simulink model "steady_state"  (R2018b)
settings: Solver=FixedStepAuto  StartTime=0.0  StopTime=0.9  FixedStep=1e-6  RelTol=1e-3
values from neighbouring files (symbols this model uses):
  J = 0.09    [dq_3hp_induction.m]
  load_time = 0.5    [dq_3hp_induction.m]
  P = 4    [dq_3hp_induction.m]
  rrp = 0.8    [dq_3hp_induction.m]
  rs = 0.45    [dq_3hp_induction.m]
  v_ll = v_rms/sqrt(3)    [dq_3hp_induction.m]
  wb = 2*pi*f    (= 376.991118431)    [dq_3hp_induction.m]
  X_lr_p = 0.75    [dq_3hp_induction.m]
  X_ls = 0.75    [dq_3hp_induction.m]
  X_M = 27    [dq_3hp_induction.m]
libraries: simulink_extras x7
settings Model: Creator=carlo  LastModifiedBy=carlo

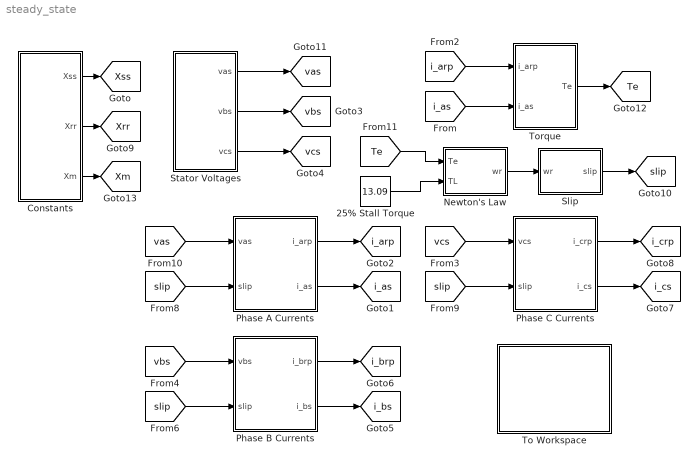
== system steady_state ==
  25% Stall Torque : Constant  Value=13.09
  Constants : Subsystem
  Newton's Law : Subsystem
  Phase A Currents : Subsystem
  Phase B Currents : Subsystem
  Phase C Currents : Subsystem
  Slip : Subsystem
  Stator Voltages : Subsystem
  To Workspace : Subsystem
  Torque : Subsystem
  tag scope: Te=global, Xm=global, Xrr=global, Xss=global, i_arp=global, i_as=global, i_brp=global, i_bs=global, i_crp=global, i_cs=global, slip=global, vas=global, vbs=global, vcs=global
  wires:
  Newton's Law/1(wr) -> Slip/1(wr)
  Slip/1(slip) -> [slip]
  [vas] -> Phase A Currents/1(vas)
  [slip] -> Phase A Currents/2(slip)
  Phase A Currents/1(i_arp) -> [i_arp]
  Phase A Currents/2(i_as) -> [i_as]
  [i_arp] -> Torque/1(i_arp)
  [i_as] -> Torque/2(i_as)
  Torque/1(Te) -> [Te]
  [Te] -> Newton's Law/1(Te)
  Stator Voltages/1(vas) -> [vas]
  Stator Voltages/2(vbs) -> [vbs]
  Stator Voltages/3(vcs) -> [vcs]
  Phase B Currents/1(i_brp) -> [i_brp]
  [slip] -> Phase B Currents/2(slip)
  Phase B Currents/2(i_bs) -> [i_bs]
  [vbs] -> Phase B Currents/1(vbs)
  Phase C Currents/1(i_crp) -> [i_crp]
  Phase C Currents/2(i_cs) -> [i_cs]
  [vcs] -> Phase C Currents/1(vcs)
  [slip] -> Phase C Currents/2(slip)
  25% Stall Torque/1 -> Newton's Law/2(TL)
  Constants/2(Xrr) -> [Xrr]
  Constants/3(Xm) -> [Xm]
  Constants/1(Xss) -> [Xss]

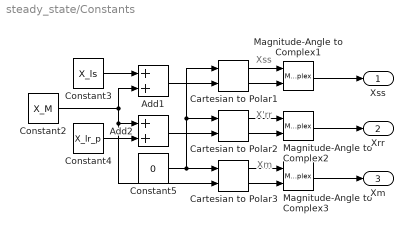
== system steady_state/Constants ==
  note: Xm
  note: X'rr
  note: Xss
  Add1 : Sum
  Add2 : Sum
  Cartesian to Polar1 : simulink_extras/Transformations/Cartesian to Polar
      settings: SourceProductName=Simulink
  Cartesian to Polar2 : simulink_extras/Transformations/Cartesian to Polar
      settings: SourceProductName=Simulink
  Cartesian to Polar3 : simulink_extras/Transformations/Cartesian to Polar
      settings: SourceProductName=Simulink
  Constant2 : Constant  Value=X_M
  Constant3 : Constant  Value=X_ls
  Constant4 : Constant  Value=X_lr_p
  Constant5 : Constant  Value=0
  Magnitude-Angle to Complex1 : MagnitudeAngleToComplex
  Magnitude-Angle to Complex2 : MagnitudeAngleToComplex
  Magnitude-Angle to Complex3 : MagnitudeAngleToComplex
  Xss : Outport
  Xrr : Outport  Port=2
  Xm : Outport  Port=3
  wires:
  Constant5/1 -> Cartesian to Polar1/1, Cartesian to Polar2/1, Cartesian to Polar3/1
  Constant2/1 -> Cartesian to Polar3/2, Add2/1, Add1/2
  Add2/1 -> Cartesian to Polar2/2
  Cartesian to Polar1/1 -> Magnitude-Angle to Complex1/1
  Add1/1 -> Cartesian to Polar1/2
  Magnitude-Angle to Complex1/1 -> Xss/1
  Constant4/1 -> Add2/2
  Cartesian to Polar1/2 -> Magnitude-Angle to Complex1/2
  Cartesian to Polar3/1 -> Magnitude-Angle to Complex3/1
  Cartesian to Polar3/2 -> Magnitude-Angle to Complex3/2
  Constant3/1 -> Add1/1
  Cartesian to Polar2/1 -> Magnitude-Angle to Complex2/1
  Cartesian to Polar2/2 -> Magnitude-Angle to Complex2/2
  Magnitude-Angle to Complex2/1 -> Xrr/1
  Magnitude-Angle to Complex3/1 -> Xm/1

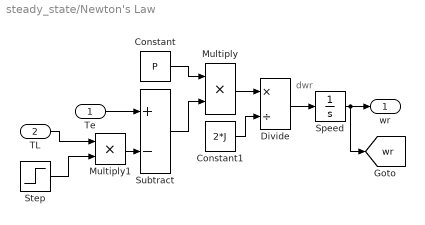
== system steady_state/Newton's Law ==
  note: dwr
  Te : Inport
  TL : Inport  Port=2
  Constant : Constant  Value=P
  Constant1 : Constant  Value=2*J
  Divide : Product  Inputs=*/
  Multiply : Product
  Multiply1 : Product
  Speed : Integrator  ContinuousStateAttributes='Speed'
  Step : Step  Time=load_time  SampleTime=0
  Subtract : Sum  Inputs=+-
  wr : Outport
  tag scope: wr=global
  wires:
  Speed/1 -> [wr], wr/1
  Multiply/1 -> Divide/1
  Constant/1 -> Multiply/1
  Divide/1 -> Speed/1
  Constant1/1 -> Divide/2
  Subtract/1 -> Multiply/2
  Te/1 -> Subtract/1
  Multiply1/1 -> Subtract/2
  TL/1 -> Multiply1/1
  Step/1 -> Multiply1/2

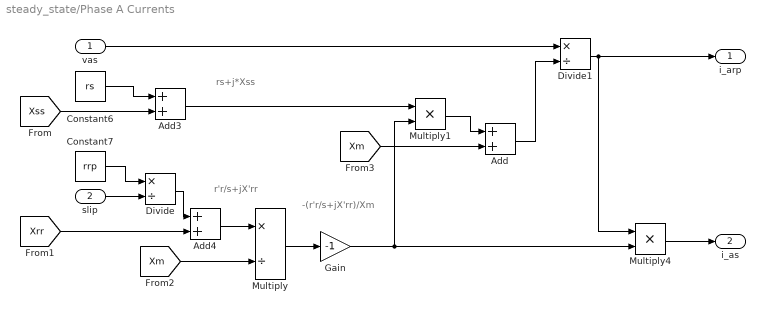
== system steady_state/Phase A Currents ==
  note: r'r/s+jX'rr
  note: rs+j*Xss
  note: -(r'r/s+jX'rr)/Xm
  vas : Inport
  slip : Inport  Port=2
  Add : Sum
  Add3 : Sum
  Add4 : Sum
  Constant6 : Constant  Value=rs
  Constant7 : Constant  Value=rrp
  Divide : Product  Inputs=*/
  Divide1 : Product  Inputs=*/
  Gain : Gain  Gain=-1
  Multiply : Product  Inputs=*/
  Multiply1 : Product
  Multiply4 : Product
  i_arp : Outport
  i_as : Outport  Port=2
  wires:
  Multiply4/1 -> i_as/1
  Multiply/1 -> Gain/1
  slip/1 -> Divide/2
  Add4/1 -> Multiply/1
  Constant7/1 -> Divide/1
  Add3/1 -> Multiply1/1
  Gain/1 -> Multiply4/2, Multiply1/2
  Divide1/1 -> i_arp/1, Multiply4/1
  Constant6/1 -> Add3/1
  vas/1 -> Divide1/1
  Add/1 -> Divide1/2
  Divide/1 -> Add4/1
  Multiply1/1 -> Add/1
  [Xrr] -> Add4/2
  [Xm] -> Multiply/2
  [Xm] -> Add/2
  [Xss] -> Add3/2

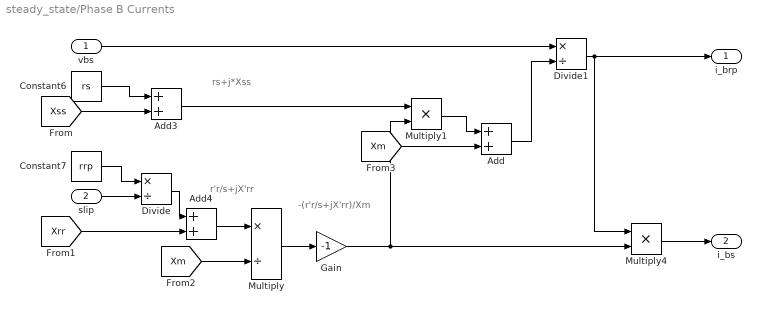
== system steady_state/Phase B Currents ==
  note: r'r/s+jX'rr
  note: rs+j*Xss
  note: -(r'r/s+jX'rr)/Xm
  vbs : Inport
  slip : Inport  Port=2
  Add : Sum
  Add3 : Sum
  Add4 : Sum
  Constant6 : Constant  Value=rs
  Constant7 : Constant  Value=rrp
  Divide : Product  Inputs=*/
  Divide1 : Product  Inputs=*/
  Gain : Gain  Gain=-1
  Multiply : Product  Inputs=*/
  Multiply1 : Product
  Multiply4 : Product
  i_brp : Outport
  i_bs : Outport  Port=2
  wires:
  Multiply4/1 -> i_bs/1
  Multiply/1 -> Gain/1
  slip/1 -> Divide/2
  Add4/1 -> Multiply/1
  Constant7/1 -> Divide/1
  Add3/1 -> Multiply1/1
  Gain/1 -> Multiply4/2, Multiply1/2
  Divide1/1 -> i_brp/1, Multiply4/1
  Constant6/1 -> Add3/1
  vbs/1 -> Divide1/1
  Add/1 -> Divide1/2
  Divide/1 -> Add4/1
  Multiply1/1 -> Add/1
  [Xss] -> Add3/2
  [Xrr] -> Add4/2
  [Xm] -> Multiply/2
  [Xm] -> Add/2

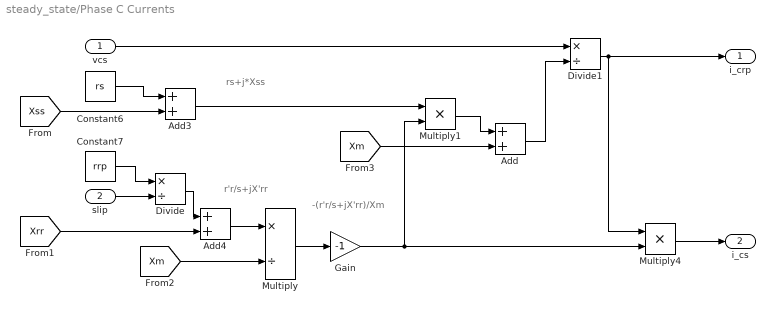
== system steady_state/Phase C Currents ==
  note: r'r/s+jX'rr
  note: rs+j*Xss
  note: -(r'r/s+jX'rr)/Xm
  vcs : Inport
  slip : Inport  Port=2
  Add : Sum
  Add3 : Sum
  Add4 : Sum
  Constant6 : Constant  Value=rs
  Constant7 : Constant  Value=rrp
  Divide : Product  Inputs=*/
  Divide1 : Product  Inputs=*/
  Gain : Gain  Gain=-1
  Multiply : Product  Inputs=*/
  Multiply1 : Product
  Multiply4 : Product
  i_crp : Outport
  i_cs : Outport  Port=2
  wires:
  Multiply4/1 -> i_cs/1
  Multiply/1 -> Gain/1
  slip/1 -> Divide/2
  Add4/1 -> Multiply/1
  Constant7/1 -> Divide/1
  Add3/1 -> Multiply1/1
  Gain/1 -> Multiply4/2, Multiply1/2
  Divide1/1 -> i_crp/1, Multiply4/1
  Constant6/1 -> Add3/1
  vcs/1 -> Divide1/1
  Add/1 -> Divide1/2
  Divide/1 -> Add4/1
  Multiply1/1 -> Add/1
  [Xss] -> Add3/2
  [Xrr] -> Add4/2
  [Xm] -> Multiply/2
  [Xm] -> Add/2

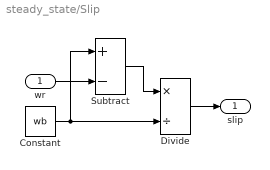
== system steady_state/Slip ==
  wr : Inport
  Constant : Constant  Value=wb
  Divide : Product  Inputs=*/
  Subtract : Sum  Inputs=+-
  slip : Outport
  wires:
  Constant/1 -> Subtract/1, Divide/2
  Subtract/1 -> Divide/1
  Divide/1 -> slip/1
  wr/1 -> Subtract/2

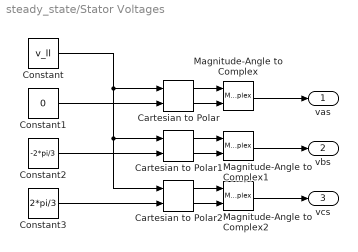
== system steady_state/Stator Voltages ==
  Cartesian to Polar : simulink_extras/Transformations/Cartesian to Polar
      settings: SourceProductName=Simulink
  Cartesian to Polar1 : simulink_extras/Transformations/Cartesian to Polar
      settings: SourceProductName=Simulink
  Cartesian to Polar2 : simulink_extras/Transformations/Cartesian to Polar
      settings: SourceProductName=Simulink
  Constant : Constant  Value=v_ll
  Constant1 : Constant  Value=0
  Constant2 : Constant  Value=-2*pi/3
  Constant3 : Constant  Value=2*pi/3
  Magnitude-Angle to Complex : MagnitudeAngleToComplex
  Magnitude-Angle to Complex1 : MagnitudeAngleToComplex
  Magnitude-Angle to Complex2 : MagnitudeAngleToComplex
  vas : Outport
  vbs : Outport  Port=2
  vcs : Outport  Port=3
  wires:
  Cartesian to Polar/1 -> Magnitude-Angle to Complex/1
  Constant2/1 -> Cartesian to Polar1/2
  Constant3/1 -> Cartesian to Polar2/2
  Constant/1 -> Cartesian to Polar2/1, Cartesian to Polar1/1, Cartesian to Polar/1
  Cartesian to Polar/2 -> Magnitude-Angle to Complex/2
  Cartesian to Polar2/1 -> Magnitude-Angle to Complex2/1
  Constant1/1 -> Cartesian to Polar/2
  Cartesian to Polar1/1 -> Magnitude-Angle to Complex1/1
  Cartesian to Polar2/2 -> Magnitude-Angle to Complex2/2
  Cartesian to Polar1/2 -> Magnitude-Angle to Complex1/2
  Magnitude-Angle to Complex/1 -> vas/1
  Magnitude-Angle to Complex2/1 -> vcs/1
  Magnitude-Angle to Complex1/1 -> vbs/1

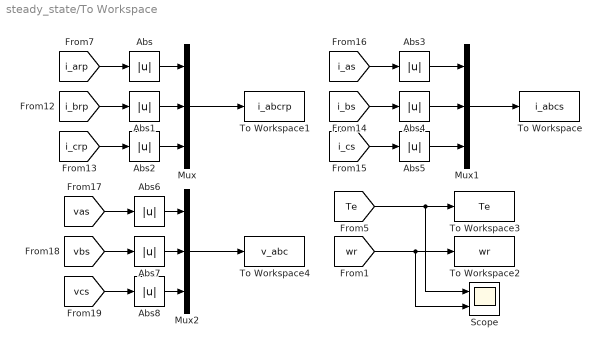
== system steady_state/To Workspace ==
  Abs{,1..8} (9 alike) : Abs
  Mux : Mux  Inputs=3
  Mux1 : Mux  Inputs=3
  Mux2 : Mux  Inputs=3
  Scope : Scope  NumInputPorts=2
  To Workspace : ToWorkspace  VariableName=i_abcs  SaveFormat=Timeseries  SampleTime=-1
  To Workspace1 : ToWorkspace  VariableName=i_abcrp  SaveFormat=Timeseries  SampleTime=-1
  To Workspace2 : ToWorkspace  VariableName=wr  SaveFormat=Timeseries  SampleTime=-1
  To Workspace3 : ToWorkspace  VariableName=Te  SaveFormat=Timeseries  SampleTime=-1
  To Workspace4 : ToWorkspace  VariableName=v_abc  SaveFormat=Timeseries  SampleTime=-1
  wires:
  Mux1/1 -> To Workspace/1
  [wr] -> Scope/2, To Workspace2/1
  Mux2/1 -> To Workspace4/1
  [Te] -> Scope/1, To Workspace3/1
  Mux/1 -> To Workspace1/1
  [i_arp] -> Abs/1
  Abs/1 -> Mux/1
  Abs1/1 -> Mux/2
  [i_brp] -> Abs1/1
  Abs2/1 -> Mux/3
  [i_crp] -> Abs2/1
  [i_as] -> Abs3/1
  Abs3/1 -> Mux1/1
  [i_bs] -> Abs4/1
  Abs4/1 -> Mux1/2
  Abs5/1 -> Mux1/3
  [i_cs] -> Abs5/1
  Abs6/1 -> Mux2/1
  [vas] -> Abs6/1
  [vbs] -> Abs7/1
  Abs8/1 -> Mux2/3
  Abs7/1 -> Mux2/2
  [vcs] -> Abs8/1

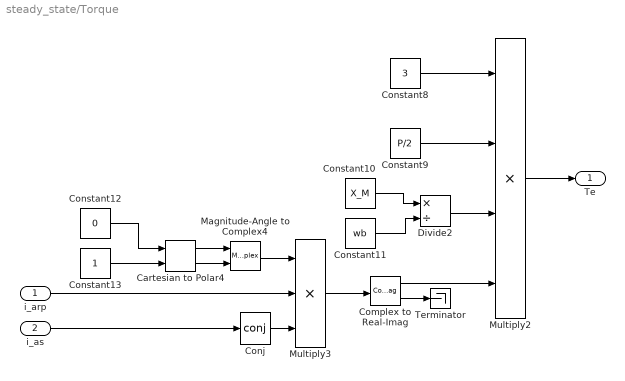
== system steady_state/Torque ==
  i_arp : Inport
  i_as : Inport  Port=2
  Cartesian to Polar4 : simulink_extras/Transformations/Cartesian to Polar
      settings: SourceProductName=Simulink
  Complex to Real-Imag : ComplexToRealImag
  Conj : Math  Operator=conj  SaturateOnIntegerOverflow=on
  Constant10 : Constant  Value=X_M
  Constant11 : Constant  Value=wb
  Constant12 : Constant  Value=0
  Constant13 : Constant
  Constant8 : Constant  Value=3
  Constant9 : Constant  Value=P/2
  Divide2 : Product  Inputs=*/
  Magnitude-Angle to Complex4 : MagnitudeAngleToComplex
  Multiply2 : Product  Inputs=****
  Multiply3 : Product  Inputs=***
  Terminator : Terminator
  Te : Outport
  wires:
  Multiply3/1 -> Complex to Real-Imag/1
  Constant12/1 -> Cartesian to Polar4/1
  Constant11/1 -> Divide2/2
  Constant8/1 -> Multiply2/1
  i_as/1 -> Conj/1
  Cartesian to Polar4/2 -> Magnitude-Angle to Complex4/2
  Constant9/1 -> Multiply2/2
  Cartesian to Polar4/1 -> Magnitude-Angle to Complex4/1
  Complex to Real-Imag/1 -> Multiply2/4
  Complex to Real-Imag/2 -> Terminator/1
  Constant10/1 -> Divide2/1
  Divide2/1 -> Multiply2/3
  Constant13/1 -> Cartesian to Polar4/2
  Magnitude-Angle to Complex4/1 -> Multiply3/1
  Conj/1 -> Multiply3/3
  Multiply2/1 -> Te/1
  i_arp/1 -> Multiply3/2
